simulink model "Simscape_Benchmark_SIM1"  (R2021a)
settings: Solver=ode45  StartTime=0.0  StopTime=PHASE.Ttotal  FixedStep=Benchmark.Sim.Tint  RelTol=1e-5  AbsTol=1e-6
undefined symbols (not defined in the file): Actuators, Analysis, antisym, Benchmark, Bus, Disturbance, FSM, IntialCond, ISOL, K_Coarse_disc_t, Kslew_opt_disc_zoh, Model, MPS, PAYLOAD, PHASE, PMA, RWIsol, RWS, SA, Sensors, Slew, slosh, thr, X, Y, Z
libraries: sm_lib x215, nesl_utility x148, simulink x65, cstblocks x36, sharedtransform x4, vrlib x3, RCTblocks x1
(part 1 of 9)
settings Model: SimulationMode=accelerator  PauseTimes=1500  Creator=Paolo  LastModifiedBy=f.sanfedino
settings SolverCC: AlgebraicLoopSolver=TrustRegion  DecoupledContinuousIntegration=on
settings DataIOCC: SignalLogging=off  DSMLogging=off  SaveTime=off
settings DebuggingCC: ReadBeforeWriteMsg=DisableAll  WriteAfterWriteMsg=DisableAll  WriteAfterReadMsg=DisableAll  AlgebraicLoopMsg=none  ArtificialAlgebraicLoopMsg=none  MaxConsecutiveZCsMsg=none  MultiTaskDSMMsg=none  UnconnectedInputMsg=none  UnconnectedOutputMsg=none  UnconnectedLineMsg=none  ModelReferenceExtraNoncontSigs=none  OperatingPointInterfaceChecksumMismatchMsg=none
settings ModelReferenceCC: UpdateModelReferenceTargets=IfOutOfDate
settings SFSimCC: SFSimEcho=off
settings DiagnosticsConfigSet: SimMechanicsInvalidVisualProperty=none  SimMechanicsCrossSectionNullEdge=none  SimMechanicsUnconnectedFramePorts=none  SimMechanicsUnconnectedGeometryPorts=none  SimMechanicsRedundantBlock=none  SimMechanicsConflictingReferenceFrames=none  SimMechanicsUnsatisfiedHighPriorityTargets=none  SimMechanicsJointTargetOverSpecification=none
settings ExplorerConfigSet: SimMechanicsOpenEditorOnUpdate=off  InternalSimMechanicsExplorerSettings="<ExplorerConfiguration><canonicalview>default</canonicalview><AnimationSetting><BasePlaybackSpeed>1.0</BasePlaybackSpeed><PlaybackSpeedFactor>1.0</PlaybackSpeedFactor></AnimationSetting><TilePanel><TileInfo><Tiles Columns=\"1\" Count=\"1\" Rows=\"1\"><Column Weight=\"1\"/><Row Weight=\"1\"/><Tile Height=\"1\" Width=\"1\" X=\"0\" Y=\"0\"/></Tiles></TileInfo><SceneInfo><SceneViewer><BGColor><R>1</R><G>1</G><B>1</B></BGColor><Camera><DoPerspective>off</DoPerspective><Position><X>3.0731714809401196</X><Y>-5.01177860946873643</Y><Z>0.913300671144394172</Z></Position><Center><X>0.412511907852218251</X><Y>-0.148244348796700232</Y><Z>-0.117628205353135465</Z></Center><Up><X>-0.119983391121796096</X><Y>0.142618601509285181</Y><Z>0.982478457961522444</Z></Up><ViewLimDist>1</ViewLimDist><YLim>1.91086627958608957</YLim><XLim>3.74866351255996477</XLim></Camera></SceneViewer></SceneInfo></TilePanel><MechEditorPanel><Cameras/><GfxPanelCameraMap/><VideoCreator><PlaybackSpeedRatio>1.0</PlaybackSpeedRatio><FrameRate>30</FrameRate><VideoFormat>Motion JPEG AVI</VideoFormat><FrameSize>auto</FrameSize></VideoCreator></MechEditorPanel></ExplorerConfiguration>"

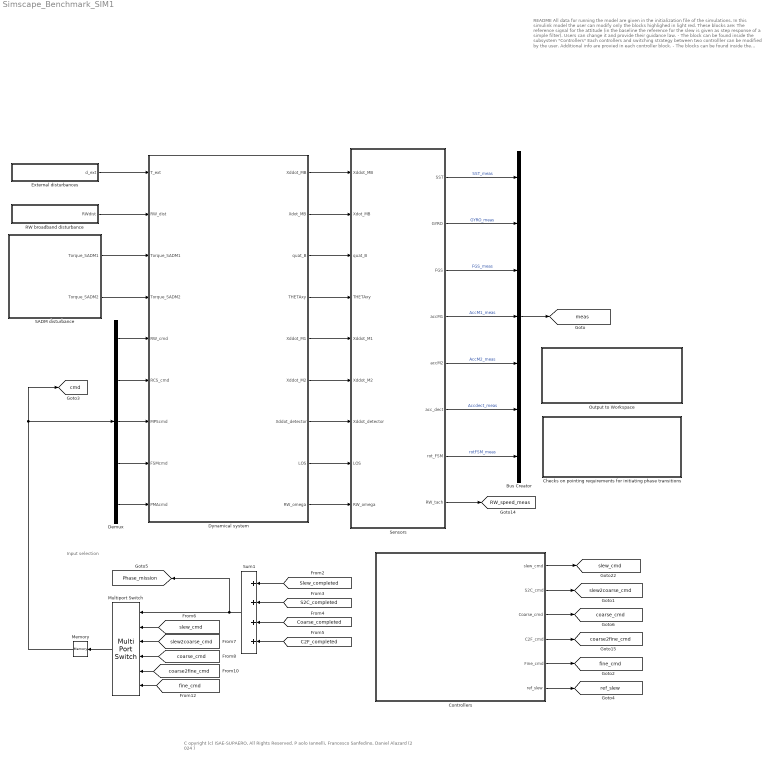
== system Simscape_Benchmark_SIM1 ==
  note: README
      |
      | All data for running the model are given in the initialization file of the simulations. In this simulink model the user can modify only the blocks highlighed in light red.
      |
      | These blocks are:
      |
      | The reference signal for the attitude (in the baseline the reference for the slew is given as step response of a simple filter). Users can change it and provide their guidance law.
      | - The block can be found inside the subsystem "Controllers"
      |
      | Each controllers and switching strategy between two controlller can be modified by the user. Additional info are provied in each controller block.
      | - The blocks can be found inside the subsystem "Controllers"
      |
      | The friction compensation algorithm can be modified by the user. A baseline one is already provided which implements a first-order filter that uses the RW tacomether measurements and the commanded torque to provide an estimate of the friction
      | - The block can be found inside the subsystem
      | "Dynamical system" -> "WEMS + Reaction wheels" -> "Friction compensation filter"
  note: Input selection
  note: C opyright (c) ISAE-SUPAERO, All Rights Reserved.
      | P aolo Iannelli, Francesco Sanfedino, Daniel Alazard (2 024 )
  Bus Creator : BusCreator  Inputs=7
  "Checks on pointing requirements for initiating phase transitions " : Subsystem
      mask Display: disp('Checks on APE req. \n for initiating \n phase transitions ')
  Controllers : Subsystem
  Demux : Demux  Outputs=[3,3,3,2,6]
  Dynamical system : Subsystem
  External disturbances : Subsystem
  Memory : Memory  InheritSampleTime=on
  Multiport Switch : MultiPortSwitch  DataPortOrder=Zero-based contiguous  Inputs=5  zeroidx=on
  Output to Workspace : Subsystem
      mask Display: disp('Output \n to \n workspace')
  RW broadband disturbance : Subsystem
  SADM disturbance : Subsystem
  Sensors : Subsystem
  Sum1 : Sum  Inputs=++++
  tag scope: Phase_mission=global, RW_speed_meas=global, cmd=global, coarse2fine_cmd=global, coarse_cmd=global, fine_cmd=global, meas=global, ref_slew=global, slew2coarse_cmd=global, slew_cmd=global
  wires:
  Dynamical system/2(Xdot_MB) -> Sensors/2(Xdot_MB)
  Bus Creator/1 -> [meas]
  Dynamical system/8(LOS) -> Sensors/8(LOS)
  Sensors/6(acc_dect) -> Bus Creator/6  "Accdect_meas"
  Sensors/7(rot_FSM) -> Bus Creator/7  "rotFSM_meas"
  Sensors/4(accM1) -> Bus Creator/4  "AccM1_meas"
  Demux/2 -> Dynamical system/6(RCS_cmd)
  Sensors/5(accM2) -> Bus Creator/5  "AccM2_meas"
  Sensors/1(SST) -> Bus Creator/1  "SST_meas"
  Demux/5 -> Dynamical system/9(PMAcmd)
  Dynamical system/7(Xddot_detector) -> Sensors/7(Xddot_detector)
  Demux/4 -> Dynamical system/8(FSMcmd)
  Sensors/2(GYRO) -> Bus Creator/2  "GYRO_meas"
  Dynamical system/4(THETAxy) -> Sensors/4(THETAxy)
  Dynamical system/5(Xddot_M1) -> Sensors/5(Xddot_M1)
  Sensors/3(FGS) -> Bus Creator/3  "FGS_meas"
  Dynamical system/3(quat_B) -> Sensors/3(quat_B)
  Demux/3 -> Dynamical system/7(MPScmd)
  Dynamical system/1(Xddot_MB) -> Sensors/1(Xddot_MB)
  Dynamical system/6(Xddot_M2) -> Sensors/6(Xddot_M2)
  Demux/1 -> Dynamical system/5(RW_cmd)
  [coarse_cmd] -> Multiport Switch/4
  [slew_cmd] -> Multiport Switch/2
  [slew2coarse_cmd] -> Multiport Switch/3
  Memory/1 -> [cmd], Demux/1
  [coarse2fine_cmd] -> Multiport Switch/5
  SADM disturbance/1(Torque_SADM1) -> Dynamical system/3(Torque_SADM1)
  SADM disturbance/2(Torque_SADM2) -> Dynamical system/4(Torque_SADM2)
  [Slew_completed] -> Sum1/1
  [S2C_completed] -> Sum1/2
  Sum1/1 -> [Phase_mission], Multiport Switch/1
  [Coarse_completed] -> Sum1/3
  [C2F_completed] -> Sum1/4
  [fine_cmd] -> Multiport Switch/6
  Multiport Switch/1 -> Memory/1
  Controllers/1(slew_cmd) -> [slew_cmd]
  Controllers/2(S2C_cmd) -> [slew2coarse_cmd]
  Controllers/3(Coarse_cmd) -> [coarse_cmd]
  Controllers/4(C2F_cmd) -> [coarse2fine_cmd]
  Controllers/5(Fine_cmd) -> [fine_cmd]
  External disturbances/1(d_ext) -> Dynamical system/1(T_ext)
  RW broadband disturbance/1(RWdist) -> Dynamical system/2(RW_dist)
  Sensors/8(RW_tach) -> [RW_speed_meas]
  Dynamical system/9(RW_omega) -> Sensors/9(RW_omega)
  Controllers/6(ref_slew) -> [ref_slew]

== system Simscape_Benchmark_SIM1/Checks on pointing requirements for initiating phase transitions  ==
  note: Coarse req. should be achieved to activate the coarse pointing phase
  note: Check for the completion of the transition phase
  note: Check for activating the transition between Slew and Coarse transient
  note: Check for the completion of the coarse pointing phaes
  note: Control to activate the transition between slew and coarse pointing
  Check Fine APE : MATLAB Function  TreatAsAtomicUnit=on  SystemSampleTime=Model.ACS_sampling.Ts
  Check coarse APE req. : MATLAB Function  TreatAsAtomicUnit=on  SystemSampleTime=Model.ACS_sampling.Ts
  Check condition for a time window (C2F) : MATLAB Function  TreatAsAtomicUnit=on  SystemSampleTime=Model.ACS_sampling.Ts
  "Check condition for a time window (S) " : MATLAB Function  TreatAsAtomicUnit=on  SystemSampleTime=Model.ACS_sampling.Ts
  Check condition for a time window (S2C) : MATLAB Function  TreatAsAtomicUnit=on  SystemSampleTime=Model.ACS_sampling.Ts
  Check slew APE req. : MATLAB Function  TreatAsAtomicUnit=on  SystemSampleTime=Model.ACS_sampling.Ts
  Constant{1,15..16,22} (4 alike) : Constant  Value=Model.ACS_sampling.Ts
  Constant12 : Constant  Value=PHASE.Coarse.REQ.APE.Value
  Constant13 : Constant  Value=Slew.RefModel.SteadyStateVector
  Constant14 : Constant  Value=PHASE.Slew.REQ.APE.Value
  Constant17 : Constant  Value=PHASE.Coarse.Duration
  Constant18 : Constant  Value=PHASE.TransitionS2C.TimeCheck
  Constant2 : Constant  Value=PHASE.Slew.TimeCheck
  Constant21 : Constant  Value=PHASE.Fine.REQ.APE.Value
  Constant23 : Constant  Value=PHASE.TransitionC2F.TimeCheck
  Constant24 : Constant  Value=Slew.RefModel.SteadyStateVector
  Constant3 : Constant  Value=PHASE.TransitionS2C.TimeCheck_reqNotMet
  Constant4 : Constant  Value=Slew.RefModel.SteadyStateVector
  Constant5 : Constant  Value=PHASE.TransitionC2F.TimeCheck_reqNotMet
  Duration of Coarse : MATLAB Function  TreatAsAtomicUnit=on  SystemSampleTime=Model.ACS_sampling.Ts
  tag scope: C2F_completed=global, CoarseAPE_notMet=global, Coarse_completed=global, FineAPE_notMet=global, S2C_completed=global, Slew_completed=global
  wires:
  Constant23/1 -> Check condition for a time window (C2F)/3(Transition_C2FtimeCheck)
  Constant1/1 -> "Check condition for a time window (S) "/2(sampling)
  [LOS] -> Check Fine APE/1(LOS)
  Duration of Coarse/1(out) -> [Coarse_completed]
  "Check condition for a time window (S) "/1(out) -> [Slew_completed]
  Constant22/1 -> Check condition for a time window (C2F)/2(sampling)
  [LOS] -> Check coarse APE req./1(LOS)
  [LOS] -> Check slew APE req./1(LOS)
  Constant2/1 -> "Check condition for a time window (S) "/3(Slew_timeCheck)
  Constant12/1 -> Check coarse APE req./3(Coarse_APEreq)
  Constant24/1 -> Check Fine APE/2(Steady_state)
  Check slew APE req./1(out) -> "Check condition for a time window (S) "/1(u)
  Check condition for a time window (C2F)/1(out) -> [C2F_completed]
  Check Fine APE/1(out) -> Check condition for a time window (C2F)/1(u)
  Constant4/1 -> Check coarse APE req./2(Steady_state)
  Constant16/1 -> Duration of Coarse/2(sampling)
  Constant15/1 -> Check condition for a time window (S2C)/2(sampling)
  Check condition for a time window (S2C)/1(out) -> [S2C_completed]
  Check coarse APE req./1(out) -> Check condition for a time window (S2C)/1(u)
  [Slew_completed] -> Check condition for a time window (S2C)/4(Slew_completed), Check coarse APE req./4(Slew_completed)
  [S2C_completed] -> Duration of Coarse/1(S2C_completed)
  Constant13/1 -> Check slew APE req./2(Steady_state)
  Constant17/1 -> Duration of Coarse/3(CoarseDuration)
  Constant21/1 -> Check Fine APE/3(Fine_APEreq)
  Constant18/1 -> Check condition for a time window (S2C)/3(Transition_S2CtimeCheck)
  Constant14/1 -> Check slew APE req./3(Slew_APEreq)
  Constant3/1 -> Check condition for a time window (S2C)/5(Transition_S2CtimeCheck_reqNotMet)
  Check condition for a time window (S2C)/2(out2) -> [CoarseAPE_notMet]
  [Coarse_completed] -> Check condition for a time window (C2F)/4(Coarse_Completed), Check Fine APE/4(Coarse_completed)
  Constant5/1 -> Check condition for a time window (C2F)/5(Transition_C2FtimeCheck_reqNotMet)
  Check condition for a time window (C2F)/2(out2) -> [FineAPE_notMet]
  [ref_signal] -> Check slew APE req./4(reference)

== system Simscape_Benchmark_SIM1/Controllers ==
  note: if value<0 no output;
      | if value>0 output of the controller
  note: COARSE TO FINE TRANSITION
  note: SLEW TO COARSE TRANSITION
  note: FINE POINTING (STEADY-STATE)
  note: SLEW CONTROLLER
  note: COARSE POINTING (STEADY-STATE)
  note: Reference attitude trajectory
  AND : Logic  AllPortsSameDT=off  OutDataTypeStr=boolean
  AND3 : Logic  AllPortsSameDT=off  OutDataTypeStr=boolean
  "Coarse 2 fine " : Subsystem
  Coarse pointing : Subsystem
  Fine pointing : Subsystem
  LTI System1 : cstblocks/LTI System  sys=Slew.Ref_model.Function_Y_disc  IC=[]
  LTI System2 : cstblocks/LTI System  sys=Slew.Ref_model.Function_Z_disc  IC=[]
  LTI System4 : cstblocks/LTI System  sys=Slew.Ref_model.Function_X_disc  IC=[]
  Mux4 : Mux  Inputs=3
  NOR : Logic  Operator=NOT  AllPortsSameDT=off  OutDataTypeStr=boolean
  NOT : Logic  Operator=NOT  AllPortsSameDT=off  OutDataTypeStr=boolean
  NOT3 : Logic  Operator=NOT  AllPortsSameDT=off  OutDataTypeStr=boolean
  Slew : Subsystem  TreatAsAtomicUnit=on
  Step4 : Step  SampleTime=Model.ACS_sampling.Ts
  TransitionSlew2Coarse : Subsystem  TreatAsAtomicUnit=on
  slew_cmd : Outport
  S2C_cmd : Outport  Port=2
  Coarse_cmd : Outport  Port=3
  C2F_cmd : Outport  Port=4
  Fine_cmd : Outport  Port=5
  ref_slew : Outport  Port=6
  tag scope: ref_signal=global
  wires:
  Step4/1 -> LTI System2/1, LTI System4/1, LTI System1/1
  AND/1 -> TransitionSlew2Coarse/3(Slew2CoarseActivation)
  [ref_signal] -> TransitionSlew2Coarse/2(ref)
  [ref_signal] -> Fine pointing/2(Input)
  [meas] -> Coarse pointing/1(meas)
  LTI System4/1 -> Mux4/1
  AND3/1 -> "Coarse 2 fine "/3(TransitionCoarse2FineActivation)
  NOR/1 -> Slew/3(slew_deactivation)
  [S2C_completed] -> NOT/1
  Mux4/1 -> ref_slew/1, [ref_signal]
  [meas] -> Fine pointing/1(meas)
  LTI System1/1 -> Mux4/2
  [Slew_completed] -> AND/1
  [meas] -> "Coarse 2 fine "/1(meas)
  Slew/1(Out1) -> slew_cmd/1
  NOT/1 -> AND/2
  [meas] -> TransitionSlew2Coarse/1(meas)
  TransitionSlew2Coarse/1(Out1) -> S2C_cmd/1
  [ref_signal] -> "Coarse 2 fine "/2(ref)
  [Slew_completed] -> NOR/1
  [Coarse_completed] -> AND3/1
  [C2F_completed] -> NOT3/1
  NOT3/1 -> AND3/2
  [ref_signal] -> Coarse pointing/2(ref)
  LTI System2/1 -> Mux4/3
  [meas] -> Slew/1(meas)
  [ref_signal] -> Slew/2(ref)
  Coarse pointing/1(<cmd>) -> Coarse_cmd/1
  "Coarse 2 fine "/1(cmd) -> C2F_cmd/1
  Fine pointing/1(cmd) -> Fine_cmd/1

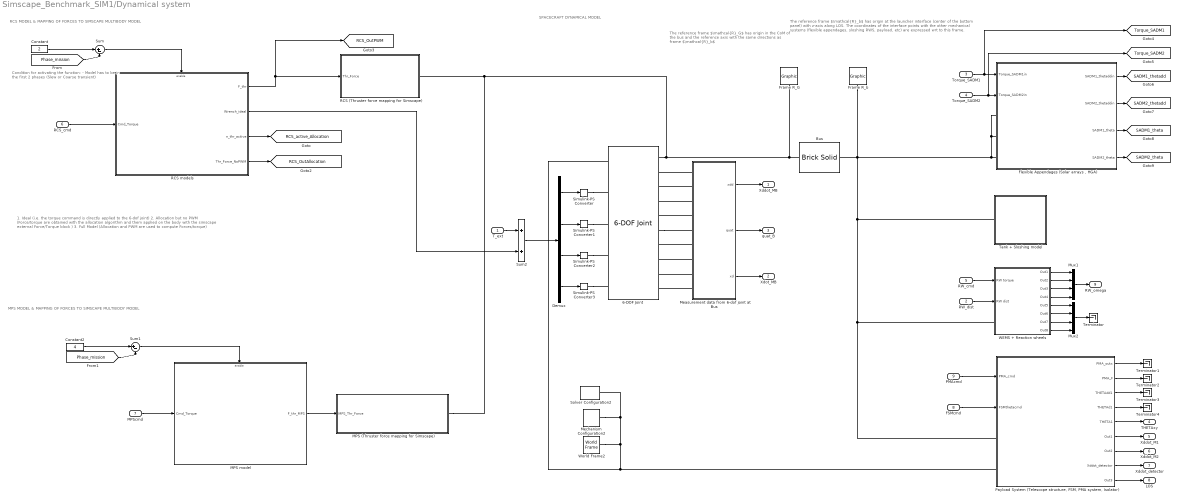
== system Simscape_Benchmark_SIM1/Dynamical system ==
  note: MPS MODEL & MAPPING OF FORCES TO SIMSCAPE MULTIBODY MODEL
  note: SPACECRAFT DYNAMICAL MODEL
  note: RCS MODEL & MAPPING OF FORCES TO SIMSCAPE MULTIBODY MODEL
  note: Condition for activating the function:
      |
      | - Model has to be in the first 2 phases (Slew or Coarse transient)
  note: 1. Ideal (i.e. the torque command is directly applied to the 6-dof joint)
      |
      | 2. Allocation but no PWM (Force/torque are obtained with the allocation algorithm and them applied on the body with the simscape external Force/Torque block )
      |
      | 3. Full Model (Allocation and PWM are used to compute Forces/torque)
  note: The reference frame $\mathcal{R}_b$ has origin at the launcher interface (center of the bottom panel) with z-axis along LOS. The coordinates of the interface points with the other mechanical systems (flexible appendages, sloshing RWS, payload, etc) are expressed wrt to this frame.
  note: The reference frame $\mathcal{R}_G$ has origin in the CoM of the bus and the reference axis with the same directions as frame $\mathcal{R}_b$
  T_ext : Inport
  RW_dist : Inport  Port=2
  Torque_SADM1 : Inport  Port=3
  Torque_SADM2 : Inport  Port=4
  RW_cmd : Inport  Port=5
  RCS_cmd : Inport  Port=6
  MPScmd : Inport  Port=7
  FSMcmd : Inport  Port=8  PortDimensions=2
  PMAcmd : Inport  Port=9
  6-DOF Joint : sm_lib/Joints/6-DOF Joint  JointMode=Normal  SenseConstraintForce=off  SenseConstraintForceX=off  SenseConstraintForceY=off  SenseConstraintForceZ=off  SenseConstraintTorque=off  SenseConstraintTorqueX=off  SenseConstraintTorqueY=off  SenseConstraintTorqueZ=off  SenseTotalForce=off  SenseTotalForceX=off  SenseTotalForceY=off  SenseTotalForceZ=off  SenseTotalTorque=off  SenseTotalTorqueX=off  SenseTotalTorqueY=off  SenseTotalTorqueZ=off  CompositeWrenchDir=FollowerOnBase  CompositeWrenchFrame=BaseFrame  PxEquilibriumPosition=0  PxEquilibriumPositionUnits=m  PxSpringStiffness=0  PxSpringStiffnessUnits=N/m  PxDampingCoefficient=0  PxDampingCoefficientUnits=N/(m/s)  PxTorqueActuationMode=InputTorque  PxMotionActuationMode=ComputedMotion  PxSensePosition=off  PxSenseVelocity=on  PxSenseAcceleration=on  PxSenseTorqueForce=off  PxSenseLowerLimitTorqueForce=off  PxSenseUpperLimitTorqueForce=off  PxLowerLimitSpecify=off  PxLowerLimitBound=-1  PxLowerLimitBoundUnits=m  PxLowerLimitStiffness=1e6  PxLowerLimitStiffnessUnits=N/m  PxLowerLimitDamping=1e3  PxLowerLimitDampingUnits=N/(m/s)  PxLowerLimitTransitionRegionWidth=1e-4  PxLowerLimitTransitionRegionWidthUnits=m  PxUpperLimitSpecify=off  PxUpperLimitBound=1  PxUpperLimitBoundUnits=m  PxUpperLimitStiffness=1e6  PxUpperLimitStiffnessUnits=N/m  PxUpperLimitDamping=1e3  PxUpperLimitDampingUnits=N/(m/s)  PxUpperLimitTransitionRegionWidth=1e-4  PxUpperLimitTransitionRegionWidthUnits=m  PxPositionTargetSpecify=off  PxPositionTargetPriority=High  PxPositionTargetValue=0  PxPositionTargetValueUnits=m  PxVelocityTargetSpecify=off  PxVelocityTargetPriority=High  PxVelocityTargetValue=0  PxVelocityTargetValueUnits=m/s  PyEquilibriumPosition=0  PyEquilibriumPositionUnits=m  PySpringStiffness=0  PySpringStiffnessUnits=N/m  PyDampingCoefficient=0  PyDampingCoefficientUnits=N/(m/s)  PyTorqueActuationMode=InputTorque  PyMotionActuationMode=ComputedMotion  PySensePosition=off  PySenseVelocity=on  PySenseAcceleration=on  PySenseTorqueForce=off  PySenseLowerLimitTorqueForce=off  PySenseUpperLimitTorqueForce=off  PyLowerLimitSpecify=off  PyLowerLimitBound=-1  PyLowerLimitBoundUnits=m  PyLowerLimitStiffness=1e6  PyLowerLimitStiffnessUnits=N/m  PyLowerLimitDamping=1e3  PyLowerLimitDampingUnits=N/(m/s)  PyLowerLimitTransitionRegionWidth=1e-4  PyLowerLimitTransitionRegionWidthUnits=m  PyUpperLimitSpecify=off  PyUpperLimitBound=1  PyUpperLimitBoundUnits=m  PyUpperLimitStiffness=1e6  PyUpperLimitStiffnessUnits=N/m  PyUpperLimitDamping=1e3  PyUpperLimitDampingUnits=N/(m/s)  PyUpperLimitTransitionRegionWidth=1e-4  PyUpperLimitTransitionRegionWidthUnits=m  PyPositionTargetSpecify=off  PyPositionTargetPriority=High  PyPositionTargetValue=0  PyPositionTargetValueUnits=m  PyVelocityTargetSpecify=off  PyVelocityTargetPriority=High  PyVelocityTargetValue=0  PyVelocityTargetValueUnits=m/s  PzEquilibriumPosition=0  PzEquilibriumPositionUnits=m  PzSpringStiffness=0  PzSpringStiffnessUnits=N/m  PzDampingCoefficient=0  PzDampingCoefficientUnits=N/(m/s)  PzTorqueActuationMode=InputTorque  PzMotionActuationMode=ComputedMotion  PzSensePosition=off  PzSenseVelocity=on  PzSenseAcceleration=on  PzSenseTorqueForce=off  PzSenseLowerLimitTorqueForce=off  PzSenseUpperLimitTorqueForce=off  PzLowerLimitSpecify=off  PzLowerLimitBound=-1  PzLowerLimitBoundUnits=m  PzLowerLimitStiffness=1e6  PzLowerLimitStiffnessUnits=N/m  PzLowerLimitDamping=1e3  PzLowerLimitDampingUnits=N/(m/s)  PzLowerLimitTransitionRegionWidth=1e-4  PzLowerLimitTransitionRegionWidthUnits=m  PzUpperLimitSpecify=off  PzUpperLimitBound=1  PzUpperLimitBoundUnits=m  PzUpperLimitStiffness=1e6  PzUpperLimitStiffnessUnits=N/m  PzUpperLimitDamping=1e3  PzUpperLimitDampingUnits=N/(m/s)  PzUpperLimitTransitionRegionWidth=1e-4  PzUpperLimitTransitionRegionWidthUnits=m  PzPositionTargetSpecify=off  PzPositionTargetPriority=High  PzPositionTargetValue=0  PzPositionTargetValueUnits=m  PzVelocityTargetSpecify=off  PzVelocityTargetPriority=High  PzVelocityTargetValue=0  PzVelocityTargetValueUnits=m/s  SphDefPosRotationMethod=None  SphDefPosRotationAngleUnits=deg  SphDefPosRotationStandardAxis=+Z  SphDefPosRotationAngle=0.0  SphDefPosRotationArbitraryAxis=[0 0 1]  SphDefPosFollAlignAxisA=+X  SphDefPosBaseAlignAxisA=+Y  SphDefPosFollAlignAxisB=+Y  SphDefPosBaseAlignAxisB=+Z  SphDefPosRotationSequenceAxes=FollowerAxes  SphDefPosRotationSequence=XYX  SphDefPosRotationSequenceAngles=[0 0 0]  SphDefPosRotationSequenceAnglesUnits=deg  SphDefPosRotationMatrix=[1 0 0; 0 1 0; 0 0 1]  SphEqPosRotationMethod=None  SphEqPosRotationAngleUnits=deg  SphEqPosRotationStandardAxis=+Z  SphEqPosRotationAngle=0.0  SphEqPosRotationArbitraryAxis=[0 0 1]  SphEqPosFollAlignAxisA=+X  SphEqPosBaseAlignAxisA=+Y  SphEqPosFollAlignAxisB=+Y  SphEqPosBaseAlignAxisB=+Z  SphEqPosRotationSequenceAxes=FollowerAxes  SphEqPosRotationSequence=XYX  SphEqPosRotationSequenceAngles=[0 0 0]  SphEqPosRotationSequenceAnglesUnits=deg  SphEqPosRotationMatrix=[1 0 0; 0 1 0; 0 0 1]  SphSpringStiffness=0  SphSpringStiffnessUnits=N*m/deg  SphDampingCoefficient=0  SphDampingCoefficientUnits=N*m/(deg/s)  SphActuateTorqueX=off  SphActuateTorqueY=off  SphActuateTorqueZ=off  SphActuateTorque=on  SphTorqueActuationMode=InputTorque  SphMotionActuationMode=ComputedMotion  SphActuationFrame=BaseFrame  SphSensePosition=on  SphSenseVelocityX=off  SphSenseVelocityY=off  SphSenseVelocityZ=off  SphSenseVelocity=on  SphSenseAccelerationX=off  SphSenseAccelerationY=off  SphSenseAccelerationZ=off  SphSenseAcceleration=on  SphSenseTorqueX=off  SphSenseTorqueY=off  SphSenseTorqueZ=off  SphSenseTorqueForce=off  SphSenseLowerLimitTorqueMag=off  SphSenseUpperLimitTorqueMag=off  SphSensingFrame=BaseFrame  SphLowerLimitSpecify=off  SphLowerLimitBound=15  SphLowerLimitBoundUnits=deg  SphLowerLimitStiffness=1e4  SphLowerLimitStiffnessUnits=N*m/deg  SphLowerLimitDamping=10  SphLowerLimitDampingUnits=N*m/(deg/s)  SphLowerLimitTransitionRegionWidth=0.1  SphLowerLimitTransitionRegionWidthUnits=deg  SphUpperLimitSpecify=off  SphUpperLimitBound=45  SphUpperLimitBoundUnits=deg  SphUpperLimitStiffness=1e4  SphUpperLimitStiffnessUnits=N*m/deg  SphUpperLimitDamping=10  SphUpperLimitDampingUnits=N*m/(deg/s)  SphUpperLimitTransitionRegionWidth=0.1  SphUpperLimitTransitionRegionWidthUnits=deg  SphPositionTargetRotationMethod=None  SphPositionTargetRotationAngleUnits=deg  SphPositionTargetRotationStandardAxis=+Z  SphPositionTargetRotationAngle=0.0  SphPositionTargetRotationArbitraryAxis=[0 0 1]  SphPositionTargetFollAlignAxisA=+X  SphPositionTargetBaseAlignAxisA=+Y  SphPositionTargetFollAlignAxisB=+Y  SphPositionTargetBaseAlignAxisB=+Z  SphPositionTargetRotationSequenceAxes=FollowerAxes  SphPositionTargetRotationSequence=XYX  SphPositionTargetRotationSequenceAngles=[0 0 0]  SphPositionTargetRotationSequenceAnglesUnits=deg  SphPositionTargetRotationMatrix=[1 0 0; 0 1 0; 0 0 1]  SphPositionTargetSpecify=off  SphPositionTargetPriority=High  SphVelocityTargetValue=[0 0 0]  SphVelocityTargetValueUnits=deg/s  SphVelocityTargetSpecify=off  SphVelocityTargetPriority=High  SphVelocityTargetInFollowerFrame=on
  Bus : sm_lib/Body Elements/Brick Solid  GraphicAmbientColor=[0.15 0.15 0.15 1.0]  BasedOnType=Density  BrickDimensions=Bus.size  BrickDimensionUnits=m  CenterOfMass=Bus.CoM_Variation_simscape  CenterOfMassUnits=m  GraphicDiffuseColor=[0.5 0.5 0.5]  Density=1000  DensityUnits=kg/m^3  DoExposeReferenceFrame=on  GraphicEmissiveColor=[0.0 0.0 0.0 1.0]  ExportEntireGeometry=off  SerializedFrames=<Frames><Frame><Id>Frame2</Id><Value><Name>F2</Name><Origin><Source>GeometricFeature</Source><FeatureName>-z surface</FeatureName></Origin><PrimaryAxis><DefinedDirection>+Z</DefinedDirection><Source>ReferenceFrame</Source><SourceDirection>+Z</SourceDirection><FeatureName></FeatureName></PrimaryAxis><SecondaryAxis><DefinedDirection>+X</DefinedDirection><Source>ReferenceFrame</Source><SourceDirection>+X</SourceDirection><FeatureName></FeatureName></SecondaryAxis></Value></Frame></Frames>  MarkerShape=Cube  MarkerSize=10  GraphicType=FromGeometry  InertiaType=Custom  Mass=Bus.m_B_SIM  MassUnits=kg  MomentsOfInertia=diag(Bus.J_B_B_SIM)'  MomentsOfInertiaUnits=kg*m^2  GraphicOpacity=0.2  ProductsOfInertia=[Bus.J_B_B_SIM(2,3) Bus.J_B_B_SIM(1,3) Bus.J_B_B_SIM(1,2)]  ProductsOfInertiaUnits=kg*m^2  GraphicShininess=75  GraphicSpecularColor=[0.5 0.5 0.5 1.0]  GraphicVisPropType=SimpleVisualProperties
  Constant : Constant  Value=2
  Constant2 : Constant  Value=4
  Demux : Demux  Outputs=[1,1,1,3]
  "Flexible Appendages (Solar arrays , HGA)" : Subsystem
      mask Display: image('$imagefile'); % Use "Edit Image" on toolstrip to change.
  Frame R_G : sm_lib/Body Elements/Graphic  GraphicType=Marker  MarkerShape=Frame  MarkerSize=30  GraphicVisPropType=SimpleVisualProperties  GraphicDiffuseColor=[1.0 0.2 0.0]  GraphicSpecularColor=[0.5 0.5 0.5 1.0]  GraphicAmbientColor=[0.15 0.15 0.15 1.0]  GraphicEmissiveColor=[0.0 0.0 0.0 1.0]  GraphicShininess=75  GraphicOpacity=0.7
  Frame R_b : sm_lib/Body Elements/Graphic  GraphicType=Marker  MarkerShape=Frame  MarkerSize=40  GraphicVisPropType=SimpleVisualProperties  GraphicDiffuseColor=[0.0 0.0 0.0]  GraphicSpecularColor=[0.5 0.5 0.5 1.0]  GraphicAmbientColor=[0.15 0.15 0.15 1.0]  GraphicEmissiveColor=[0.0 0.0 0.0 1.0]  GraphicShininess=75  GraphicOpacity=0.7
  MPS (Thruster force mapping for Simscape) : Subsystem
  MPS model : Subsystem  TreatAsAtomicUnit=on
  Measurement data from 6-dof joint at Bus : Subsystem
  Mechanism Configuration2 : sm_lib/Utilities/Mechanism Configuration  UniformGravity=None  GravityVector=[0 0 -9.8]  GravityVectorUnits=m/s^2  GravityUnits=m/s^2  LinearizationDelta=1e-25  JointModeTransitionNonlinearIterations=2
  Mux1 : Mux
  Mux2 : Mux
  "Payload System (Telescope structure, FSM, PMA system, Isolator)" : Subsystem
      mask Display: image('$imagefile'); % Use "Edit Image" on toolstrip to change.
  RCS (Thruster force mapping for Simscape) : Subsystem
  RCS models : Subsystem  TreatAsAtomicUnit=on
  Simulink-PS Converter{,1..3} (4 alike) : nesl_utility/Simulink-PS Converter  PhysicalDomain=network_engine_domain  SubClassName=ps_input  LeftPortType=input  RightPortType=output  PseudoPeriodic=off  Frequencies=[]  NoiseDistribution=none  NoiseParameters=[]  Unit=1  AffineConversion=off  FilteringAndDerivatives=provide  SimscapeFilterOrder=1  InputFilterTimeConstant=0.001  UdotUserProvided=0
      settings: SourceProductBaseCode=PW,SS
  Solver Configuration2 : nesl_utility/Solver Configuration  PhysicalDomain=network_engine_domain  SubClassName=solver  LeftPortType=input  RightPortType=generic  Tones=[]  Harmonics=[]  SimulateNoise=off  Profile=off  UseLocalSampling=off  EnableSwitchedLinearOptims=on  FrequencyDomain=off  UseCCode=off  RelTol=0.001  AbsTol=1e-06  MinStep=1e-09  ToWorkspace=off  RevertToSquareIcSolve=off  NumHomotopyIterations=100  PhasorMode=off  PhasorModeNumHarmonics=1  DoDC=off  ResidualTolerance=1e-8  UseLocalSolver=off  LocalSolverChoice=NE_BACKWARD_EULER_ADVANCER  LocalSolverSampleTime=0.001  DoFixedCost=off  MaxNonlinIter=3  MaxModeIter=2  ComputeImpulses=off  ImpulseIterations=2  LinearAlgebra=auto  EquationFormulation=NE_TIME_EF  DelaysMemoryBudget=1024  AutomaticFiltering=off  FilteringTimeConstant=0.001  PartitionStorageMethod=AS_NEEDED  PartitionMemoryBudget=1024  PartitionMethod=ROBUST
      settings: SourceProductBaseCode=PW,SS
  Sum : Sum  Inputs=|+-
  Sum1 : Sum  Inputs=|+-
  Sum2 : Sum
  Tank + Sloshing model : Subsystem
      mask Display: image('$imagefile'); % Use "Edit Image" on toolstrip to change.
  Terminator{,1..4} (5 alike) : Terminator
  WEMS + Reaction wheels : Subsystem
      mask Display: image('$imagefile'); % Use "Edit Image" on toolstrip to change.
  World Frame2 : sm_lib/Frames and Transforms/World Frame
  Xddot_MB : Outport
  Xdot_MB : Outport  Port=2
  quat_B : Outport  Port=3
  THETAxy : Outport  Port=4
  Xddot_M1 : Outport  Port=5
  Xddot_M2 : Outport  Port=6
  Xddot_detector : Outport  Port=7
  LOS : Outport  Port=8
  RW_omega : Outport  Port=9
  tag scope: RCS_OutAllocation=global, RCS_OutPWM=global, RCS_active_Allocation=global, SADM1_theta=global, SADM1_thetadd=global, SADM2_theta=global, SADM2_thetadd=global, Torque_SADM1=global, Torque_SADM2=global
  wires:
  WEMS + Reaction wheels/3(Out3) -> Mux1/3
  WEMS + Reaction wheels/5(Out5) -> Mux2/1
  "Payload System (Telescope structure, FSM, PMA system, Isolator)"/6(Out1) -> Xddot_M1/1
  "Payload System (Telescope structure, FSM, PMA system, Isolator)"/7(Out2) -> Xddot_M2/1
  RW_cmd/1 -> WEMS + Reaction wheels/1(RW torque)
  Mux2/1 -> Terminator/1
  Demux/1 -> Simulink-PS Converter/1
  "Payload System (Telescope structure, FSM, PMA system, Isolator)"/1(PMA_outx) -> Terminator1/1
  "Payload System (Telescope structure, FSM, PMA system, Isolator)"/5(THETA1) -> THETAxy/1
  WEMS + Reaction wheels/7(Out7) -> Mux2/3
  WEMS + Reaction wheels/8(Out8) -> Mux2/4
  WEMS + Reaction wheels/2(Out2) -> Mux1/2
  Torque_SADM2/1 -> [Torque_SADM2], "Flexible Appendages (Solar arrays , HGA)"/2(Torque_SADM2in)
  WEMS + Reaction wheels/4(Out4) -> Mux1/4
  Torque_SADM1/1 -> [Torque_SADM1], "Flexible Appendages (Solar arrays , HGA)"/1(Torque_SADM1in)
  FSMcmd/1 -> "Payload System (Telescope structure, FSM, PMA system, Isolator)"/2(FSMthetacmd)
  RW_dist/1 -> WEMS + Reaction wheels/2(RW dist)
  "Payload System (Telescope structure, FSM, PMA system, Isolator)"/3(THETAdd1) -> Terminator3/1
  Mux1/1 -> RW_omega/1
  WEMS + Reaction wheels/1(Out1) -> Mux1/1
  "Payload System (Telescope structure, FSM, PMA system, Isolator)"/4(THETAd1) -> Terminator4/1
  WEMS + Reaction wheels/6(Out6) -> Mux2/2
  "Payload System (Telescope structure, FSM, PMA system, Isolator)"/2(PMA_F) -> Terminator2/1
  PMAcmd/1 -> "Payload System (Telescope structure, FSM, PMA system, Isolator)"/1(PMA_cmd)
  Demux/4 -> Simulink-PS Converter3/1
  Demux/2 -> Simulink-PS Converter1/1
  Demux/3 -> Simulink-PS Converter2/1
  "Flexible Appendages (Solar arrays , HGA)"/1(SADM1_thetaddin) -> [SADM1_thetadd]
  "Flexible Appendages (Solar arrays , HGA)"/2(SADM2_thetaddin) -> [SADM2_thetadd]
  "Flexible Appendages (Solar arrays , HGA)"/3(SADM1_theta) -> [SADM1_theta]
  "Flexible Appendages (Solar arrays , HGA)"/4(SADM2_theta) -> [SADM2_theta]
  "Payload System (Telescope structure, FSM, PMA system, Isolator)"/8(Xddot_detector) -> Xddot_detector/1
  "Payload System (Telescope structure, FSM, PMA system, Isolator)"/9(Out3) -> LOS/1
  Sum2/1 -> Demux/1
  T_ext/1 -> Sum2/1
  Measurement data from 6-dof joint at Bus/1(xdd) -> Xddot_MB/1
  Measurement data from 6-dof joint at Bus/2(quat) -> quat_B/1
  Measurement data from 6-dof joint at Bus/3(xd) -> Xdot_MB/1
  RCS_cmd/1 -> RCS models/1(Cmd_Torque)
  RCS models/2(Wrench_ideal) -> Sum2/2
  [Phase_mission] -> Sum/2
  Constant/1 -> Sum/1
  Sum/1 -> RCS models/Enable
  RCS models/3(n_thr_active) -> [RCS_active_Allocation]
  RCS models/1(F_thr) -> [RCS_OutPWM], RCS (Thruster force mapping for Simscape)/1(Thr_Force)
  RCS models/4(Thr_Force_NoPWM) -> [RCS_OutAllocation]
  Sum1/1 -> MPS model/Enable
  Constant2/1 -> Sum1/1
  [Phase_mission] -> Sum1/2
  MPScmd/1 -> MPS model/1(Cmd_Torque)
  MPS model/1(F_thr_MPS) -> MPS (Thruster force mapping for Simscape)/1(MPS_Thr_Force)
  connections:
  Frame R_b/RConn1 -- "Flexible Appendages (Solar arrays , HGA)"/LConn1 -- "Flexible Appendages (Solar arrays , HGA)"/LConn2 -- "Flexible Appendages (Solar arrays , HGA)"/LConn3 -- "Payload System (Telescope structure, FSM, PMA system, Isolator)"/LConn1 -- WEMS + Reaction wheels/LConn1 -- Tank + Sloshing model/LConn1 -- Bus/LConn1
  Simulink-PS Converter/RConn1 -- 6-DOF Joint/LConn2
  Simulink-PS Converter2/RConn1 -- 6-DOF Joint/LConn4
  Simulink-PS Converter1/RConn1 -- 6-DOF Joint/LConn3
  Simulink-PS Converter3/RConn1 -- 6-DOF Joint/LConn5
  6-DOF Joint/LConn1 -- "Payload System (Telescope structure, FSM, PMA system, Isolator)"/LConn2 -- Solver Configuration2/RConn1 -- Mechanism Configuration2/RConn1 -- World Frame2/RConn1
  Bus/RConn1 -- 6-DOF Joint/RConn1 -- RCS (Thruster force mapping for Simscape)/RConn1 -- MPS (Thruster force mapping for Simscape)/RConn1 -- Frame R_G/RConn1
  Measurement data from 6-dof joint at Bus/LConn1 -- 6-DOF Joint/RConn2
  Measurement data from 6-dof joint at Bus/LConn2 -- 6-DOF Joint/RConn3
  Measurement data from 6-dof joint at Bus/LConn3 -- 6-DOF Joint/RConn4
  Measurement data from 6-dof joint at Bus/LConn4 -- 6-DOF Joint/RConn5
  6-DOF Joint/RConn6 -- Measurement data from 6-dof joint at Bus/LConn5
  Measurement data from 6-dof joint at Bus/LConn6 -- 6-DOF Joint/RConn7
  Measurement data from 6-dof joint at Bus/LConn7 -- 6-DOF Joint/RConn8
  Measurement data from 6-dof joint at Bus/LConn8 -- 6-DOF Joint/RConn9
  Measurement data from 6-dof joint at Bus/LConn9 -- 6-DOF Joint/RConn10

== system Simscape_Benchmark_SIM1/External disturbances ==
  Constant : Constant  Value=[0;0;0]
  Disturbance.External.SelectSim : Gain  Gain=Disturbance.External.SelectSim
  Mux1 : Mux  Inputs=[3,3]
  Mux3 : Mux  Inputs=3
  Sine Wave1 : Sin  Amplitude=Disturbance.External.Value(1)  Frequency=Disturbance.External.FreqSin  Phase=pi/2  SampleTime=0
  Sine Wave2 : Sin  Amplitude=Disturbance.External.Value(2)  Frequency=Disturbance.External.FreqSin  Phase=pi/2  SampleTime=0
  Sine Wave3 : Sin  Amplitude=Disturbance.External.Value(3)  Frequency=Disturbance.External.FreqSin  Phase=pi/2  SampleTime=0
  d_ext : Outport
  wires:
  Constant/1 -> Mux1/1
  Mux1/1 -> [dist_ext], d_ext/1
  Sine Wave1/1 -> Mux3/1
  Sine Wave3/1 -> Mux3/3
  Mux3/1 -> Disturbance.External.SelectSim/1
  Sine Wave2/1 -> Mux3/2
  Disturbance.External.SelectSim/1 -> Mux1/2
